simulink model "capacitor1"  (R2013a)
settings: Solver=ode4  StartTime=0.0  StopTime=0.1  FixedStep=1e-6  RelTol=1e-3
values from neighbouring files (symbols this model uses):
  Lload = Xload/wout_fund    [acemp_sixth.m]    (also in immd_base_varyingmod.m = Xload/wout; immd_design_elen.m = Xload/wout; immd_efficiency.m = Xload/wout; immd_simulation_base.m = Xload/wout)
  ma = 1    [IMMD_design_tool_v01.m]    (also in IMMD_design_tool_v02.m = 0.9; immd_base_varyingmod.m; immd_design_elen.m = 0.8; immd_efficiency.m = 0.85)
  Rload = Zload*pf    [acemp_sixth.m]    (also in immd_base_varyingmod.m; immd_design_elen.m; immd_efficiency.m; immd_simulation_base.m)
  wout = 2*pi*fout    (= 314.159265359)    [immd_base_varyingmod.m]    (also in immd_design_elen.m; immd_efficiency.m; immd_simulation_base.m)
libraries: powerlib x27, powerlib_meascontrol x6
settings Model: Creator=ugurm  LastModifiedBy=ugurm

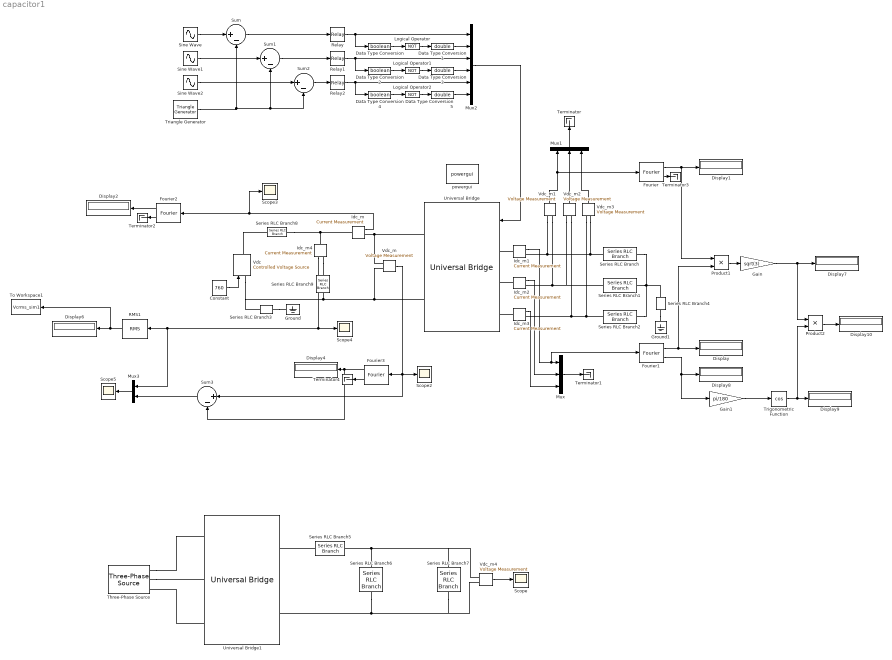
== system capacitor1 ==
  Constant : Constant  Value=760
  Data Type Conversion : DataTypeConversion  OutDataTypeStr=boolean
  Data Type Conversion1 : DataTypeConversion  OutDataTypeStr=double
  Data Type Conversion2 : DataTypeConversion  OutDataTypeStr=boolean
  Data Type Conversion3 : DataTypeConversion  OutDataTypeStr=double
  Data Type Conversion4 : DataTypeConversion  OutDataTypeStr=boolean
  Data Type Conversion5 : DataTypeConversion  OutDataTypeStr=double
  Display{,1..2,4,6..10} (9 alike) : Display
      Display7 settings: Format=short_e
  Fourier : powerlib_meascontrol/Measurements/Fourier  Freq=fout  n=1  InInit=[0, 0]  Ts=0
  Fourier1 : powerlib_meascontrol/Measurements/Fourier  Freq=fout  n=1  InInit=[0, 0]  Ts=0
  Fourier2 : powerlib_meascontrol/Measurements/Fourier  Freq=fout  n=0  InInit=[0, 0]  Ts=0
  Fourier3 : powerlib_meascontrol/Measurements/Fourier  Freq=fout  n=0  InInit=[0, 0]  Ts=0
  Gain : Gain  Gain=sqrt(3)
  Gain1 : Gain  Gain=pi/180
  Ground : powerlib/Elements/Ground  LConnTagsString=a
  Ground1 : powerlib/Elements/Ground  LConnTagsString=a
  Idc_m{,1..4} (5 alike) : powerlib/Measurements/Current Measurement  PhasorSimulation=off  OutputType=Complex  PSBequivalent=0
  Logical Operator : Logic  Operator=NOT  AllPortsSameDT=off  OutDataTypeStr=boolean
  Logical Operator1 : Logic  Operator=NOT  AllPortsSameDT=off  OutDataTypeStr=boolean
  Logical Operator2 : Logic  Operator=NOT  AllPortsSameDT=off  OutDataTypeStr=boolean
  Mux : Mux  Inputs=3
  Mux1 : Mux  Inputs=3
  Mux2 : Mux  Inputs=6
  Mux3 : Mux  Inputs=2
  Product1 : Product
  Product2 : Product
  RMS1 : powerlib_meascontrol/Measurements/RMS  TrueRMS=on  Freq=50  RMSInit=120  Ts=0
  Relay : Relay
  Relay1 : Relay
  Relay2 : Relay
  Scope{,2..5} (5 alike) : Scope
      Scope2 settings: YMin=475  YMax=975  SaveName=ScopeData2
      Scope3 settings: YMin=500  YMax=800  SaveName=ScopeData3
      Scope4 settings: YMin=500  YMax=800  SaveName=ScopeData4
      Scope5 settings: YMin=-250  YMax=225  SaveName=ScopeData5
  Series RLC Branch : powerlib/Elements/Series RLC Branch  LConnTagsString=__new0  RConnTagsString=__new0  BranchType=RL  Resistance=Rload  Inductance=Lload  SetiL0=off  InitialCurrent=0  Capacitance=1e-6  Setx0=off  InitialVoltage=0  Measurements=None
  Series RLC Branch1 : powerlib/Elements/Series RLC Branch  LConnTagsString=__new0  RConnTagsString=__new0  BranchType=RL  Resistance=Rload  Inductance=Lload  SetiL0=off  InitialCurrent=0  Capacitance=1e-6  Setx0=off  InitialVoltage=0  Measurements=None
  Series RLC Branch2 : powerlib/Elements/Series RLC Branch  LConnTagsString=__new0  RConnTagsString=__new0  BranchType=RL  Resistance=Rload  Inductance=Lload  SetiL0=off  InitialCurrent=0  Capacitance=1e-6  Setx0=off  InitialVoltage=0  Measurements=None
  Series RLC Branch3 : powerlib/Elements/Series RLC Branch  LConnTagsString=__new0  RConnTagsString=__new0  BranchType=R  Resistance=1e12  Inductance=Lload  SetiL0=off  InitialCurrent=0  Capacitance=1e-6  Setx0=off  InitialVoltage=0  Measurements=None
  Series RLC Branch4 : powerlib/Elements/Series RLC Branch  LConnTagsString=__new0  RConnTagsString=__new0  BranchType=R  Resistance=1e12  Inductance=Lload  SetiL0=off  InitialCurrent=0  Capacitance=1e-6  Setx0=off  InitialVoltage=0  Measurements=None
  Series RLC Branch5 : powerlib/Elements/Series RLC Branch  LConnTagsString=__new0  RConnTagsString=__new0  BranchType=L  Resistance=1e12  Inductance=3e-3  SetiL0=off  InitialCurrent=0  Capacitance=1e-6  Setx0=off  InitialVoltage=0  Measurements=None
  Series RLC Branch6 : powerlib/Elements/Series RLC Branch  LConnTagsString=__new0  RConnTagsString=__new0  BranchType=C  Resistance=1e12  Inductance=Lload  SetiL0=off  InitialCurrent=0  Capacitance=3e-3  Setx0=off  InitialVoltage=0  Measurements=None
  Series RLC Branch7 : powerlib/Elements/Series RLC Branch  LConnTagsString=__new0  RConnTagsString=__new0  BranchType=R  Resistance=25  Inductance=Lload  SetiL0=off  InitialCurrent=0  Capacitance=1e-6  Setx0=off  InitialVoltage=0  Measurements=None
  Series RLC Branch8 : powerlib/Elements/Series RLC Branch  LConnTagsString=__new0  RConnTagsString=__new0  BranchType=R  Resistance=5  Inductance=Lload  SetiL0=off  InitialCurrent=0  Capacitance=1e-6  Setx0=off  InitialVoltage=0  Measurements=None
  Series RLC Branch9 : powerlib/Elements/Series RLC Branch  LConnTagsString=__new0  RConnTagsString=__new0  BranchType=C  Resistance=1e12  Inductance=Lload  SetiL0=off  InitialCurrent=0  Capacitance=10e-6  Setx0=off  InitialVoltage=0  Measurements=None
  Sine Wave : Sin  Amplitude=ma  Frequency=wout  SampleTime=0
  Sine Wave1 : Sin  Amplitude=ma  Frequency=wout  Phase=-2*pi/3  SampleTime=0
  Sine Wave2 : Sin  Amplitude=ma  Frequency=wout  Phase=2*pi/3  SampleTime=0
  Sum{,1..3} (4 alike) : Sum  Inputs=|+-
  Terminator{,1..4} (5 alike) : Terminator
  Three-Phase Source : powerlib/Electrical Sources/Three-Phase Source  Voltage=500  PhaseAngle=0  Frequency=50  InternalConnection=Yg  SpecifyImpedance=off  Resistance=0  Inductance=0  ShortCircuitLevel=100e6  BaseVoltage=500  XRratio=7  BusType=swing  Pref=0  Qref=0  Qmin=-inf  Qmax=inf
  To Workspace1 : ToWorkspace  VariableName=Vcrms_sim1  SampleTime=-1
  Triangle Generator : powerlib_meascontrol/Pulse & Signal Generators/Triangle Generator  Freq=fsw  Phase=0  Ts=1e-6
  Trigonometric Function : Trigonometry  Operator=cos
  Universal Bridge : powerlib/Power Electronics/Universal Bridge  Arms=3  SnubberResistance=1e5  SnubberCapacitance=inf  Device=IGBT / Diodes  Ron=1e-6  Lon=0  ForwardVoltages="[  0  0  ]"  ForwardVoltage=0  GTOparameters=[ 10e-6 , 20e-6 ]  IGBTparameters=[ 1e-6 , 2e-6 ]  Measurements=None  Measurements_2=None  converterType=Rectifier
  Universal Bridge1 : powerlib/Power Electronics/Universal Bridge  Arms=3  SnubberResistance=1e5  SnubberCapacitance=inf  Device=Diodes  Ron=1e-6  Lon=0  ForwardVoltages="[  0  0  ]"  ForwardVoltage=0  GTOparameters=[ 10e-6 , 20e-6 ]  IGBTparameters=[ 1e-6 , 2e-6 ]  Measurements=None  Measurements_2=None  converterType=Rectifier
  Vdc : powerlib/Electrical Sources/Controlled Voltage Source  Initialize=off  Source_Type=DC  Amplitude=200  Phase=0  Frequency=0  Measurements=None
  Vdc_m{,1..4} (5 alike) : powerlib/Measurements/Voltage Measurement  PhasorSimulation=off  OutputType=Complex  PSBequivalent=0
  powergui : powerlib/powergui  Priority=1  SimulationMode=Discrete  SolverType=Tustin  SampleTime=1e-6  frequency=60  SPID=off  DisableSnubberDevices=off  DisableRonSwitches=off  DisableVfSwitches=off  SwTol=0  Interpol=off  DisplayEquations=off  frequencyindice=0  Pbase=100e6  ErrMax=1e-4  Iterations=50  UnitsV=kV  UnitsW=MW  FunctionMessages=off  echomessages=off  HookPort=off  EnableUseOfTLC=off  x0status=blocks  RestoreLinks=warning  ResistiveCurrentMeasurement=off  Frange=[0:2:500]  Ylog=off  Xlog=on  ShowGrid=off  save=off  variable=ZData  structure=idc  ZoomFFT=off  StartTime=0.1  cycles=20  DisplayStyle=5  fundamental=50  FreqAxis=off  MaxFrequency=20000  frequencyindicesteady=1  RmsSteady=1  display=off  Ts=0  methode=off
  wires:
  Constant/1 -> Vdc/1
  Idc_m/1 -> Scope3/1, Fourier2/1
  Idc_m1/1 -> Fourier1/1, Mux/1
  Idc_m2/1 -> Mux/2
  Idc_m3/1 -> Mux/3
  Mux/1 -> Terminator1/1
  Sine Wave/1 -> Sum/1
  Triangle Generator/1 -> Sum1/2, Sum2/2, Sum/2
  Sine Wave1/1 -> Sum1/1
  Sine Wave2/1 -> Sum2/1
  Sum/1 -> Relay/1
  Sum1/1 -> Relay1/1
  Sum2/1 -> Relay2/1
  Data Type Conversion/1 -> Logical Operator/1
  Relay/1 -> Data Type Conversion/1, Mux2/1
  Logical Operator/1 -> Data Type Conversion1/1
  Data Type Conversion1/1 -> Mux2/2
  Data Type Conversion2/1 -> Logical Operator1/1
  Relay1/1 -> Data Type Conversion2/1, Mux2/3
  Logical Operator1/1 -> Data Type Conversion3/1
  Data Type Conversion3/1 -> Mux2/4
  Data Type Conversion4/1 -> Logical Operator2/1
  Relay2/1 -> Data Type Conversion4/1, Mux2/5
  Logical Operator2/1 -> Data Type Conversion5/1
  Data Type Conversion5/1 -> Mux2/6
  Mux2/1 -> Universal Bridge/1
  Fourier1/1 -> Display/1, Product1/2
  Vdc_m1/1 -> Mux1/1, Fourier/1
  Vdc_m2/1 -> Mux1/2
  Vdc_m3/1 -> Mux1/3
  Fourier/1 -> Product1/1, Display1/1
  Fourier2/1 -> Display2/1
  Product1/1 -> Gain/1
  Gain/1 -> Product2/1, Display7/1
  Fourier1/2 -> Display8/1, Gain1/1
  Trigonometric Function/1 -> Product2/2, Display9/1
  Gain1/1 -> Trigonometric Function/1
  Product2/1 -> Display10/1
  Mux1/1 -> Terminator/1
  Fourier2/2 -> Terminator2/1
  Fourier/2 -> Terminator3/1
  Vdc_m/1 -> Sum3/1, Fourier3/1, Scope2/1
  Vdc_m4/1 -> Scope/1
  Fourier3/1 -> Sum3/2, Display4/1
  Fourier3/2 -> Terminator4/1
  Idc_m4/1 -> Scope4/1, Mux3/1, RMS1/1
  RMS1/1 -> To Workspace1/1, Display6/1
  Sum3/1 -> Mux3/2
  Mux3/1 -> Scope5/1
  connections:
  Universal Bridge/RConn1 -- Vdc_m/LConn1 -- Idc_m/RConn1
  Universal Bridge/RConn2 -- Vdc_m/LConn2 -- Vdc/LConn1 -- Series RLC Branch3/LConn1 -- Series RLC Branch9/RConn1
  Idc_m1/LConn1 -- Universal Bridge/LConn1
  Idc_m2/LConn1 -- Universal Bridge/LConn2
  Idc_m3/LConn1 -- Universal Bridge/LConn3
  Vdc_m3/LConn1 -- Series RLC Branch2/LConn1 -- Vdc_m2/LConn2 -- Idc_m3/RConn1
  Series RLC Branch1/LConn1 -- Vdc_m2/LConn1 -- Vdc_m1/LConn2 -- Idc_m2/RConn1
  Series RLC Branch/LConn1 -- Vdc_m3/LConn2 -- Vdc_m1/LConn1 -- Idc_m1/RConn1
  Series RLC Branch/RConn1 -- Series RLC Branch4/LConn1 -- Series RLC Branch2/RConn1 -- Series RLC Branch1/RConn1
  Series RLC Branch3/RConn1 -- Ground/LConn1
  Series RLC Branch4/RConn1 -- Ground1/LConn1
  Three-Phase Source/RConn2 -- Universal Bridge1/LConn2
  Three-Phase Source/RConn1 -- Universal Bridge1/LConn1
  Universal Bridge1/LConn3 -- Three-Phase Source/RConn3
  Series RLC Branch5/RConn1 -- Universal Bridge1/RConn1
  Series RLC Branch6/LConn1 -- Vdc_m4/LConn1 -- Series RLC Branch7/LConn1 -- Series RLC Branch5/LConn1
  Series RLC Branch6/RConn1 -- Vdc_m4/LConn2 -- Series RLC Branch7/RConn1 -- Universal Bridge1/RConn2
  Series RLC Branch8/LConn1 -- Idc_m4/LConn1 -- Idc_m/LConn1
  Idc_m4/RConn1 -- Series RLC Branch9/LConn1
  Series RLC Branch8/RConn1 -- Vdc/RConn1
